simulink model "prystupalab8_si"  (R2023b)
settings: Solver=VariableStepAuto  StartTime=0.0  StopTime=10.0  RelTol=1e-3
values from neighbouring files (symbols this model uses):
  A = [-a1/A1 a1/A1; a1/A2 -(a1+a2)/A2]    [prystupalab8.m]
  B = [1/A1 0; 0 1/A2]    [prystupalab8.m]
  C = [1,0;0,1]    [prystupalab8.m]
  D = [0,0;0,0]    [prystupalab8.m]
  dfw1 = 0.1*fwmax1    [prystupalab8.m]
  dfw2 = 0    [prystupalab8.m]
  fw1 = tabFw1(i)    [prystupalab8.m]
  fw2 = 0.1*fwmax2    [prystupalab8.m]
  H0 = [H01 H02]    [prystupalab8.m]
  t0 = 10    [prystupalab8.m]
settings Model: Creator=Adam  LastModifiedBy=Adam

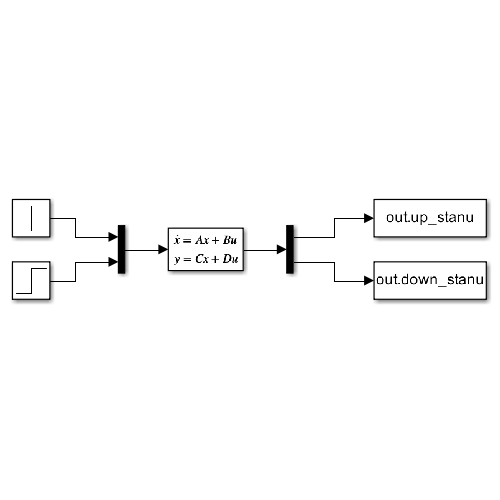
[thumbnail: Simulink's stored preview of the top-level diagram]
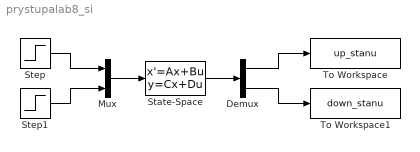
== system prystupalab8_si ==
  Demux : Demux  Outputs=2
  Mux : Mux  Inputs=2
  State-Space : StateSpace  A=A  B=B  C=C  D=D  InitialCondition=H0
  Step : Step  Time=t0  Before=fw1  After=fw1+dfw1  SampleTime=0
  Step1 : Step  Time=t0  Before=fw2  After=fw2+dfw2  SampleTime=0
  To Workspace : ToWorkspace  VariableName=up_stanu  SampleTime=-1
  To Workspace1 : ToWorkspace  VariableName=down_stanu  SampleTime=-1
  wires:
  Step/1 -> Mux/1
  Step1/1 -> Mux/2
  Mux/1 -> State-Space/1
  State-Space/1 -> Demux/1
  Demux/1 -> To Workspace/1
  Demux/2 -> To Workspace1/1
